simulink model "pi_OfflineRL_H2DF_2023a"  (R2023a)
settings: Solver=FixedStepAuto  StartTime=0.0  StopTime=inf  FixedStep=0.001  RelTol=1e-3  EnableMultiTasking=on
values from neighbouring files (symbols this model uses):
  C2C_NMPC = init_C2C_NMPC_H2DF(C2C_NMPC.expdata)    [init_pi_OfflineRL_H2DF_2023a.m]
  LowerLimit = ([0.17e-3;350;-2;2e-3] - C2C_NMPC.Normalization.controls.mean)./(C2C_NMPC.Normalization.controls.std)    [init_pi_OfflineRL_H2DF_2023a.m]
  UpperLimit = ([0.5e-3;900;10;5.5e-3] - C2C_NMPC.Normalization.controls.mean)./(C2C_NMPC.Normalization.controls.std)    [init_pi_OfflineRL_H2DF_2023a.m]
undefined symbols (not defined in the file or in its folder): DiscIntNeverNeededParam
libraries: deeplib x9, rllib x3, raspberrypiNetworklib x1
(part 3 of 4)

== system pi_OfflineRL_H2DF_2023a/main_C2C/main_C2C_RL/RL_Controller/Subsystem ==
  note: 1:TD3
      | 2:PPO
  Refernce : Inport
  Outputs : Inport  Port=2
  Enable : Inport  Port=3
  LSTM States : Inport  Port=4
  If : If
  If Action Subsystem : Subsystem  TreatAsAtomicUnit=on
  If Action Subsystem1 : Subsystem  TreatAsAtomicUnit=on
  Merge : Merge
  Selector3 : Selector  IndexOptions=Index vector (dialog)  Indices=[5:8]  OutputSizes=1
  Observation : Outport
  wires:
  Selector3/1 -> If Action Subsystem/1(Reference)
  LSTM States/1 -> If Action Subsystem/3(LSTM States)
  Refernce/1 -> Selector3/1
  Outputs/1 -> If Action Subsystem/2(Outputs)
  Enable/1 -> If/1
  If/1 -> If Action Subsystem/Action
  If/2 -> If Action Subsystem1/Action
  If Action Subsystem/1(observations) -> Merge/1
  If Action Subsystem1/1(observations) -> Merge/2
  Merge/1 -> Observation/1

== system pi_OfflineRL_H2DF_2023a/main_C2C/main_C2C_RL/post_processing/ denormalizing reference ==
  IMEP_norm : Inport
  NOX_norm : Inport  Port=2
  soot_norm : Inport  Port=3
  MPRR_norm : Inport  Port=4
  Constant : Constant  Value=C2C_NMPC.Normalization.outputs.mean(1)
  Constant1 : Constant  Value=C2C_NMPC.Normalization.outputs.mean(2)
  Constant2 : Constant  Value=C2C_NMPC.Normalization.outputs.mean(3)
  Constant3 : Constant  Value=C2C_NMPC.Normalization.outputs.mean(4)
  Gain : Gain  Gain=C2C_NMPC.Normalization.outputs.std(1)
  Gain1 : Gain  Gain=C2C_NMPC.Normalization.outputs.std(2)
  Gain2 : Gain  Gain=C2C_NMPC.Normalization.outputs.std(3)
  Gain3 : Gain  Gain=C2C_NMPC.Normalization.outputs.std(4)
  Sum{1..3,5} (4 alike) : Sum  Inputs=|++
  IMEP : Outport
  NOX : Outport  Port=2
  soot : Outport  Port=3
  MPRR : Outport  Port=4
  wires:
  Gain/1 -> Sum5/1
  IMEP_norm/1 -> Gain/1
  Constant/1 -> Sum5/2
  Sum5/1 -> IMEP/1
  Gain1/1 -> Sum1/1
  Constant1/1 -> Sum1/2
  NOX_norm/1 -> Gain1/1
  Sum1/1 -> NOX/1
  Gain2/1 -> Sum2/1
  Constant2/1 -> Sum2/2
  soot_norm/1 -> Gain2/1
  Sum2/1 -> soot/1
  Gain3/1 -> Sum3/1
  Constant3/1 -> Sum3/2
  MPRR_norm/1 -> Gain3/1
  Sum3/1 -> MPRR/1

== system pi_OfflineRL_H2DF_2023a/main_C2C/main_C2C_RL/post_processing/Subsystem ==
  controller_ status : Inport
  LSTM_States : Inport  Port=2
  Selector2 : Selector  IndexOptions=Index vector (dialog)  Indices=[1:(C2C_NMPC.Dims.n_hidden_states+ C2C_NMPC.Dims.n_cell_states)]  OutputSizes=1
  Selector3 : Selector  IndexOptions=Index vector (dialog)  Indices=[41:56]  OutputSizes=1
  Subtract : Sum  Inputs=+-
  Out1 : Outport
  wires:
  Selector3/1 -> Subtract/1
  Selector2/1 -> Subtract/2
  controller_ status/1 -> Selector3/1
  Subtract/1 -> Out1/1
  LSTM_States/1 -> Selector2/1

== system pi_OfflineRL_H2DF_2023a/main_C2C/main_C2C_RL/post_processing/Subsystem1 ==
  controller_ status : Inport
  Last_Output_MC : Inport  Port=2
  " denormalizing reference" : Subsystem
  Demux : Demux
  Mux : Mux
  Mux1 : Mux  Inputs=2
  Mux2 : Mux
  Selector1 : Selector  IndexOptions=Index vector (dialog)  Indices=[(4 + C2C_NMPC.Dims.n_controls * C2C_NMPC.Opts.N + 1 * (C2C_NMPC.Dims.n_states) + C2C_NMPC.Dims.n_LSTM_states + C2C_NMPC.Dims.n_controls +1):( 4 + C2C_NMPC.Dims.n_controls * C2C_NMPC.Opts.N + 2* C2C_NMPC.Dims.n_states)]  OutputSizes=1
  Selector2 : Selector  IndexOptions=Index vector (dialog)  Indices=[(4 + C2C_NMPC.Dims.n_controls * C2C_NMPC.Opts.N + 2 * (C2C_NMPC.Dims.n_states) + C2C_NMPC.Dims.n_LSTM_states + C2C_NMPC.Dims.n_controls +1):( 4 + C2C_NMPC.Dims.n_controls * C2C_NMPC.Opts.N + 3* C2C_NMPC.Dims.n_states)]  OutputSizes=1
  Selector3 : Selector  IndexOptions=Index vector (dialog)  Indices=[(4 + C2C_NMPC.Dims.n_controls * C2C_NMPC.Opts.N + 1* (C2C_NMPC.Dims.n_LSTM_states + C2C_NMPC.Dims.n_controls) +1) : (4 + C2C_NMPC.Dims.n_controls * C2C_NMPC.Opts.N + 1* C2C_NMPC.Dims.n_states)]  OutputSizes=1
  Selector4 : Selector  IndexOptions=Index vector (dialog)  Indices=[(4 + C2C_NMPC.Dims.n_controls * C2C_NMPC.Opts.N + 3 * (C2C_NMPC.Dims.n_states) + C2C_NMPC.Dims.n_LSTM_states + C2C_NMPC.Dims.n_controls +1):( 4 + C2C_NMPC.Dims.n_controls * C2C_NMPC.Opts.N + 4* C2C_NMPC.Dims.n_states)]  OutputSizes=1
  Subsystem : Subsystem
  Out1 : Outport
  wires:
  Last_Output_MC/1 -> Demux/1
  controller_ status/1 -> Selector4/1, Selector2/1, Selector1/1, Selector3/1
  Mux1/1 -> Out1/1
  Mux/1 -> Mux1/2
  Demux/1 -> " denormalizing reference"/1(IMEP_norm)
  Demux/2 -> " denormalizing reference"/2(NOX_norm)
  Demux/3 -> " denormalizing reference"/3(soot_norm)
  Demux/4 -> " denormalizing reference"/4(MPRR_norm)
  " denormalizing reference"/2(NOX) -> Mux2/2
  " denormalizing reference"/1(IMEP) -> Mux2/1
  " denormalizing reference"/3(soot) -> Mux2/3
  " denormalizing reference"/4(MPRR) -> Mux2/4
  Mux2/1 -> Mux1/1
  Subsystem/1(Node_0) -> Mux/1
  Selector3/1 -> Subsystem/1(In1)
  Selector1/1 -> Subsystem/2(In2)
  Subsystem/2(Node_1) -> Mux/2
  Subsystem/3(Node_2) -> Mux/3
  Subsystem/4(Node_3) -> Mux/4
  Selector4/1 -> Subsystem/4(In4)
  Selector2/1 -> Subsystem/3(In3)

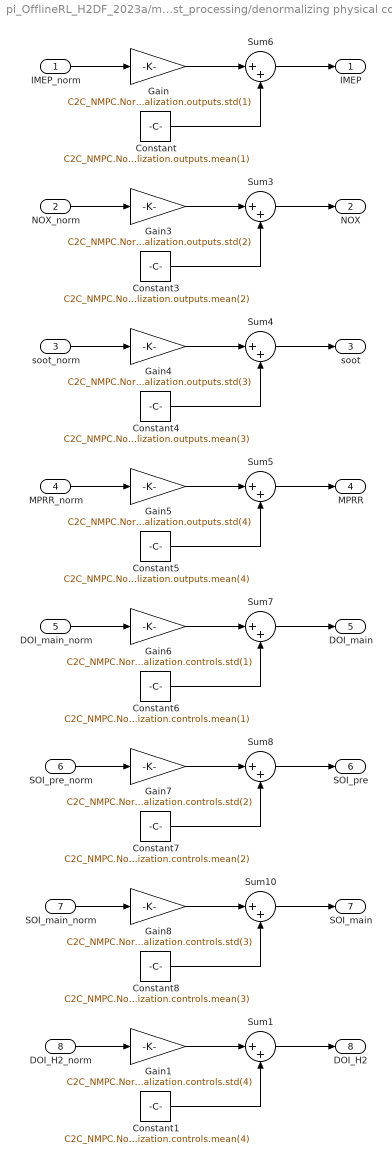
== system pi_OfflineRL_H2DF_2023a/main_C2C/main_C2C_RL/post_processing/denormalizing physical controls and outputs ==
  IMEP_norm : Inport
  NOX_norm : Inport  Port=2
  soot_norm : Inport  Port=3
  MPRR_norm : Inport  Port=4
  DOI_main_norm : Inport  Port=5
  SOI_pre_norm : Inport  Port=6
  SOI_main_norm : Inport  Port=7
  DOI_H2_norm : Inport  Port=8
  Constant : Constant  Value=C2C_NMPC.Normalization.outputs.mean(1)
  Constant1 : Constant  Value=C2C_NMPC.Normalization.controls.mean(4)
  Constant3 : Constant  Value=C2C_NMPC.Normalization.outputs.mean(2)
  Constant4 : Constant  Value=C2C_NMPC.Normalization.outputs.mean(3)
  Constant5 : Constant  Value=C2C_NMPC.Normalization.outputs.mean(4)
  Constant6 : Constant  Value=C2C_NMPC.Normalization.controls.mean(1)
  Constant7 : Constant  Value=C2C_NMPC.Normalization.controls.mean(2)
  Constant8 : Constant  Value=C2C_NMPC.Normalization.controls.mean(3)
  Gain : Gain  Gain=C2C_NMPC.Normalization.outputs.std(1)
  Gain1 : Gain  Gain=C2C_NMPC.Normalization.controls.std(4)
  Gain3 : Gain  Gain=C2C_NMPC.Normalization.outputs.std(2)
  Gain4 : Gain  Gain=C2C_NMPC.Normalization.outputs.std(3)
  Gain5 : Gain  Gain=C2C_NMPC.Normalization.outputs.std(4)
  Gain6 : Gain  Gain=C2C_NMPC.Normalization.controls.std(1)
  Gain7 : Gain  Gain=C2C_NMPC.Normalization.controls.std(2)
  Gain8 : Gain  Gain=C2C_NMPC.Normalization.controls.std(3)
  Sum{1,3..8,10} (8 alike) : Sum  Inputs=|++
  IMEP : Outport
  NOX : Outport  Port=2
  soot : Outport  Port=3
  MPRR : Outport  Port=4
  DOI_main : Outport  Port=5
  SOI_pre : Outport  Port=6
  SOI_main : Outport  Port=7
  DOI_H2 : Outport  Port=8
  wires:
  Gain4/1 -> Sum4/1
  Constant3/1 -> Sum3/2
  Constant4/1 -> Sum4/2
  Gain3/1 -> Sum3/1
  Constant5/1 -> Sum5/2
  Gain5/1 -> Sum5/1
  Constant/1 -> Sum6/2
  Sum3/1 -> NOX/1
  NOX_norm/1 -> Gain3/1
  Sum5/1 -> MPRR/1
  Gain/1 -> Sum6/1
  IMEP_norm/1 -> Gain/1
  Sum6/1 -> IMEP/1
  MPRR_norm/1 -> Gain5/1
  Sum4/1 -> soot/1
  soot_norm/1 -> Gain4/1
  Constant7/1 -> Sum8/2
  Gain8/1 -> Sum10/1
  Constant6/1 -> Sum7/2
  Gain7/1 -> Sum8/1
  Sum10/1 -> SOI_main/1
  DOI_main_norm/1 -> Gain6/1
  Sum7/1 -> DOI_main/1
  Gain6/1 -> Sum7/1
  Sum8/1 -> SOI_pre/1
  Constant8/1 -> Sum10/2
  SOI_main_norm/1 -> Gain8/1
  SOI_pre_norm/1 -> Gain7/1
  Sum1/1 -> DOI_H2/1
  Constant1/1 -> Sum1/2
  Gain1/1 -> Sum1/1
  DOI_H2_norm/1 -> Gain1/1

== system pi_OfflineRL_H2DF_2023a/main_C2C/main_C2C_RL/pre_processing1/normalize_last_outputs_MC ==
  data_in : Inport
  Constant : Constant  Value=C2C_NMPC.Normalization.outputs.mean(1)
  Constant1 : Constant  Value=C2C_NMPC.Normalization.outputs.mean(2)
  Constant2 : Constant  Value=C2C_NMPC.Normalization.outputs.mean(3)
  Constant3 : Constant  Value=C2C_NMPC.Normalization.outputs.mean(4)
  Demux : Demux
  Gain : Gain  Gain=1/C2C_NMPC.Normalization.outputs.std(1)
  Gain1 : Gain  Gain=1/C2C_NMPC.Normalization.outputs.std(2)
  Gain2 : Gain  Gain=1/C2C_NMPC.Normalization.outputs.std(3)
  Gain3 : Gain  Gain=1/C2C_NMPC.Normalization.outputs.std(4)
  Mux : Mux
  Selector1 : Selector  IndexOptions=Index vector (dialog)  Indices=[1:4]  OutputSizes=1
  Sum{1..3,5} (4 alike) : Sum  Inputs=|+-
  last_outputs_MC : Outport  VectorParamsAs1DForOutWhenUnconnected=off
  wires:
  Demux/2 -> Sum1/1
  Constant2/1 -> Sum2/2
  Sum2/1 -> Gain2/1
  Sum1/1 -> Gain1/1
  Gain3/1 -> Mux/4
  Gain1/1 -> Mux/2
  Constant1/1 -> Sum1/2
  Demux/3 -> Sum2/1
  Gain2/1 -> Mux/3
  Mux/1 -> last_outputs_MC/1
  Constant3/1 -> Sum3/2
  Sum3/1 -> Gain3/1
  Gain/1 -> Mux/1
  Sum5/1 -> Gain/1
  Constant/1 -> Sum5/2
  Demux/1 -> Sum5/1
  data_in/1 -> Selector1/1
  Demux/4 -> Sum3/1
  Selector1/1 -> Demux/1

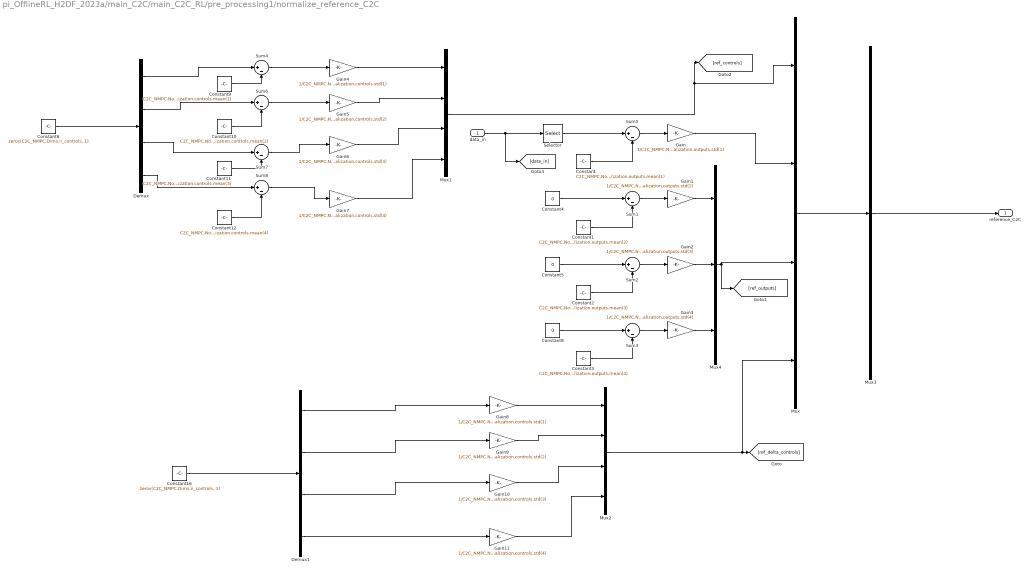
== system pi_OfflineRL_H2DF_2023a/main_C2C/main_C2C_RL/pre_processing1/normalize_reference_C2C ==
  data_in : Inport
  Constant : Constant  Value=C2C_NMPC.Normalization.outputs.mean(1)
  Constant1 : Constant  Value=C2C_NMPC.Normalization.outputs.mean(2)
  Constant10 : Constant  Value=C2C_NMPC.Normalization.controls.mean(2)
  Constant11 : Constant  Value=C2C_NMPC.Normalization.controls.mean(3)
  Constant12 : Constant  Value=C2C_NMPC.Normalization.controls.mean(4)
  Constant16 : Constant  Value=zeros(C2C_NMPC.Dims.n_controls, 1)
  Constant2 : Constant  Value=C2C_NMPC.Normalization.outputs.mean(3)
  Constant3 : Constant  Value=C2C_NMPC.Normalization.outputs.mean(4)
  Constant4 : Constant  Value=0
  Constant5 : Constant  Value=0
  Constant6 : Constant  Value=zeros(C2C_NMPC.Dims.n_controls, 1)
  Constant8 : Constant  Value=0
  Constant9 : Constant  Value=C2C_NMPC.Normalization.controls.mean(1)
  Demux : Demux
  Demux1 : Demux
  Gain : Gain  Gain=1/C2C_NMPC.Normalization.outputs.std(1)
  Gain1 : Gain  Gain=1/C2C_NMPC.Normalization.outputs.std(2)
  Gain10 : Gain  Gain=1/C2C_NMPC.Normalization.controls.std(3)
  Gain11 : Gain  Gain=1/C2C_NMPC.Normalization.controls.std(4)
  Gain2 : Gain  Gain=1/C2C_NMPC.Normalization.outputs.std(3)
  Gain3 : Gain  Gain=1/C2C_NMPC.Normalization.outputs.std(4)
  Gain4 : Gain  Gain=1/C2C_NMPC.Normalization.controls.std(1)
  Gain5 : Gain  Gain=1/C2C_NMPC.Normalization.controls.std(2)
  Gain6 : Gain  Gain=1/C2C_NMPC.Normalization.controls.std(3)
  Gain7 : Gain  Gain=1/C2C_NMPC.Normalization.controls.std(4)
  Gain8 : Gain  Gain=1/C2C_NMPC.Normalization.controls.std(1)
  Gain9 : Gain  Gain=1/C2C_NMPC.Normalization.controls.std(2)
  Mux : Mux
  Mux1 : Mux
  Mux2 : Mux
  Mux3 : Mux  Inputs=1
  Mux4 : Mux  Inputs=3
  Selector : Selector  IndexOptions=Index vector (dialog)  Indices=[5]  OutputSizes=1
  Sum{1..8} (8 alike) : Sum  Inputs=|+-
  reference_C2C : Outport  VectorParamsAs1DForOutWhenUnconnected=off
  wires:
  Constant/1 -> Sum5/2
  data_in/1 -> [data_in], Selector/1
  Sum5/1 -> Gain/1
  Selector/1 -> Sum5/1
  Constant4/1 -> Sum1/1
  Sum1/1 -> Gain1/1
  Constant1/1 -> Sum1/2
  Constant5/1 -> Sum2/1
  Sum2/1 -> Gain2/1
  Constant2/1 -> Sum2/2
  Constant8/1 -> Sum3/1
  Sum3/1 -> Gain3/1
  Constant3/1 -> Sum3/2
  Demux/1 -> Sum4/1
  Sum4/1 -> Gain4/1
  Constant9/1 -> Sum4/2
  Constant6/1 -> Demux/1
  Demux/2 -> Sum6/1
  Constant10/1 -> Sum6/2
  Sum6/1 -> Gain5/1
  Gain5/1 -> Mux1/2
  Gain4/1 -> Mux1/1
  Sum7/1 -> Gain6/1
  Constant11/1 -> Sum7/2
  Demux/3 -> Sum7/1
  Constant12/1 -> Sum8/2
  Sum8/1 -> Gain7/1
  Demux/4 -> Sum8/1
  Gain7/1 -> Mux1/4
  Gain6/1 -> Mux1/3
  Gain9/1 -> Mux2/2
  Gain11/1 -> Mux2/4
  Constant16/1 -> Demux1/1
  Gain8/1 -> Mux2/1
  Gain10/1 -> Mux2/3
  Demux1/4 -> Gain11/1
  Demux1/3 -> Gain10/1
  Demux1/2 -> Gain9/1
  Demux1/1 -> Gain8/1
  Mux2/1 -> [ref_delta_controls], Mux/4
  Mux3/1 -> reference_C2C/1
  Mux/1 -> Mux3/1
  Gain1/1 -> Mux4/1
  Gain2/1 -> Mux4/2
  Gain3/1 -> Mux4/3
  Gain/1 -> Mux/2
  Mux4/1 -> Mux/3, [ref_outputs]
  Mux1/1 -> [ref_controls], Mux/1

== system pi_OfflineRL_H2DF_2023a/main_C2C_RL/RL_Controller/RL_Controller_ifAction/RL_Controller_PPO1 ==
  In : Inport
  Action Port : ActionPort  ActionPortLabel=case [ 3 ]:
  Data Type Conversion1 : DataTypeConversion  OutDataTypeStr=single  SaturateOnIntegerOverflow=off  RndMeth=Floor
  Predict1 : deeplib/Predict  Network=Network from MAT-file  NetworkFunction=squeezenet  NetworkFilePath=C:\GIT\sharma_ma_rlonh2df\acados_implementation\rl\Results\20240912\Agent.mat  MiniBatchSize=128  InputDataFormats={ 'input_1', 'BC' }  Predictions=on  Activations={}  ForceInterpretedSim=off  EnableDLNetwork=on
  Reshape : Reshape  OutputDimensionality=Row vector (2-D)
  Selector1 : Selector  IndexOptions=Index vector (dialog)  Indices=[13:16]  OutputSizes=1
  Selector2 : Selector  IndexOptions=Index vector (dialog)  Indices=[17:24]  OutputSizes=1
  Selector3 : Selector  IndexOptions=Index vector (dialog)  Indices=[1:12]  OutputSizes=1
  Selector4 : Selector  IndexOptions=Index vector (dialog)  Indices=[25]  OutputSizes=1
  Subsystem : Subsystem
  Control_norm_NN_params : Outport
  wires:
  Predict1/1 -> Control_norm_NN_params/1
  Reshape/1 -> Predict1/1
  Data Type Conversion1/1 -> Reshape/1
  Subsystem/1(Observation) -> Data Type Conversion1/1
  In/1 -> Selector3/1, Selector1/1, Selector4/1, Selector2/1
  Selector3/1 -> Subsystem/1(Refernce)
  Selector1/1 -> Subsystem/2(Outputs)
  Selector2/1 -> Subsystem/3(LSTM States)
  Selector4/1 -> Subsystem/4(Enable)

== system pi_OfflineRL_H2DF_2023a/main_C2C_RL/RL_Controller/RL_Controller_ifAction/RL_Controller_PPO2 ==
  In : Inport
  Action Port : ActionPort  ActionPortLabel=case [ 4 ]:
  Data Type Conversion1 : DataTypeConversion  OutDataTypeStr=single  SaturateOnIntegerOverflow=off  RndMeth=Floor
  Predict1 : deeplib/Predict  Network=Network from MAT-file  NetworkFunction=squeezenet  NetworkFilePath=C:\GIT\sharma_ma_rlonh2df\acados_implementation\rl\Results\2024095\Agent.mat  MiniBatchSize=128  InputDataFormats={ 'input_1', 'BC' }  Predictions=on  Activations={}  ForceInterpretedSim=off  EnableDLNetwork=on
  Reshape : Reshape  OutputDimensionality=Row vector (2-D)
  Selector1 : Selector  IndexOptions=Index vector (dialog)  Indices=[13:16]  OutputSizes=1
  Selector2 : Selector  IndexOptions=Index vector (dialog)  Indices=[17:24]  OutputSizes=1
  Selector3 : Selector  IndexOptions=Index vector (dialog)  Indices=[1:12]  OutputSizes=1
  Selector4 : Selector  IndexOptions=Index vector (dialog)  Indices=[25]  OutputSizes=1
  Subsystem : Subsystem
  Control_norm_NN_params : Outport
  wires:
  Predict1/1 -> Control_norm_NN_params/1
  Reshape/1 -> Predict1/1
  Data Type Conversion1/1 -> Reshape/1
  Subsystem/1(Observation) -> Data Type Conversion1/1
  In/1 -> Selector3/1, Selector1/1, Selector4/1, Selector2/1
  Selector3/1 -> Subsystem/1(Refernce)
  Selector1/1 -> Subsystem/2(Outputs)
  Selector2/1 -> Subsystem/3(LSTM States)
  Selector4/1 -> Subsystem/4(Enable)

== system pi_OfflineRL_H2DF_2023a/main_C2C_RL/RL_Controller/RL_Controller_ifAction/RL_Controller_PPO3 ==
  In : Inport
  Action Port : ActionPort  ActionPortLabel=case [ 5 ]:
  Data Type Conversion1 : DataTypeConversion  OutDataTypeStr=single  SaturateOnIntegerOverflow=off  RndMeth=Floor
  Predict1 : deeplib/Predict  Network=Network from MAT-file  NetworkFunction=squeezenet  NetworkFilePath=C:\GIT\sharma_ma_rlonh2df\acados_implementation\rl\Results\2024097\Agent.mat  MiniBatchSize=128  InputDataFormats={ 'input_1', 'BC' }  Predictions=on  Activations={}  ForceInterpretedSim=off  EnableDLNetwork=on
  Reshape : Reshape  OutputDimensionality=Row vector (2-D)
  Selector1 : Selector  IndexOptions=Index vector (dialog)  Indices=[13:16]  OutputSizes=1
  Selector2 : Selector  IndexOptions=Index vector (dialog)  Indices=[17:24]  OutputSizes=1
  Selector3 : Selector  IndexOptions=Index vector (dialog)  Indices=[1:12]  OutputSizes=1
  Selector4 : Selector  IndexOptions=Index vector (dialog)  Indices=[25]  OutputSizes=1
  Subsystem : Subsystem
  Control_norm_NN_params : Outport
  wires:
  Predict1/1 -> Control_norm_NN_params/1
  Reshape/1 -> Predict1/1
  Data Type Conversion1/1 -> Reshape/1
  Subsystem/1(Observation) -> Data Type Conversion1/1
  In/1 -> Selector3/1, Selector1/1, Selector4/1, Selector2/1
  Selector3/1 -> Subsystem/1(Refernce)
  Selector1/1 -> Subsystem/2(Outputs)
  Selector2/1 -> Subsystem/3(LSTM States)
  Selector4/1 -> Subsystem/4(Enable)

== system pi_OfflineRL_H2DF_2023a/main_C2C_RL/RL_Controller/RL_Controller_ifAction/RL_Controller_PPO4 ==
  In : Inport
  Action Port : ActionPort  ActionPortLabel=case [ 6 ]:
  Data Type Conversion1 : DataTypeConversion  OutDataTypeStr=single  SaturateOnIntegerOverflow=off  RndMeth=Floor
  Predict1 : deeplib/Predict  Network=Network from MAT-file  NetworkFunction=squeezenet  NetworkFilePath=C:\GIT\sharma_ma_rlonh2df\acados_implementation\rl\Results\2024098\Agent.mat  MiniBatchSize=128  InputDataFormats={ 'input_1', 'BC' }  Predictions=on  Activations={}  ForceInterpretedSim=off  EnableDLNetwork=on
  Reshape : Reshape  OutputDimensionality=Row vector (2-D)
  Selector1 : Selector  IndexOptions=Index vector (dialog)  Indices=[13:16]  OutputSizes=1
  Selector2 : Selector  IndexOptions=Index vector (dialog)  Indices=[17:24]  OutputSizes=1
  Selector3 : Selector  IndexOptions=Index vector (dialog)  Indices=[1:12]  OutputSizes=1
  Selector4 : Selector  IndexOptions=Index vector (dialog)  Indices=[25]  OutputSizes=1
  Subsystem : Subsystem
  Control_norm_NN_params : Outport
  wires:
  Predict1/1 -> Control_norm_NN_params/1
  Reshape/1 -> Predict1/1
  Data Type Conversion1/1 -> Reshape/1
  Subsystem/1(Observation) -> Data Type Conversion1/1
  In/1 -> Selector3/1, Selector1/1, Selector4/1, Selector2/1
  Selector3/1 -> Subsystem/1(Refernce)
  Selector1/1 -> Subsystem/2(Outputs)
  Selector2/1 -> Subsystem/3(LSTM States)
  Selector4/1 -> Subsystem/4(Enable)

== system pi_OfflineRL_H2DF_2023a/main_C2C_RL/RL_Controller/RL_Controller_ifAction/RL_Controller_PPO5 ==
  In : Inport
  Action Port : ActionPort  ActionPortLabel=case [ 1 ]:
  Data Type Conversion1 : DataTypeConversion  OutDataTypeStr=single  SaturateOnIntegerOverflow=off  RndMeth=Floor
  Predict1 : deeplib/Predict  Network=Network from MAT-file  NetworkFunction=squeezenet  NetworkFilePath=C:\GIT\sharma_ma_rlonh2df\acados_implementation\rl\Results\20240909\Agent.mat  MiniBatchSize=128  InputDataFormats={ 'input_1', 'BC' }  Predictions=on  Activations={}  ForceInterpretedSim=off  EnableDLNetwork=on
  Reshape : Reshape  OutputDimensionality=Row vector (2-D)
  Selector1 : Selector  IndexOptions=Index vector (dialog)  Indices=[13:16]  OutputSizes=1
  Selector2 : Selector  IndexOptions=Index vector (dialog)  Indices=[17:24]  OutputSizes=1
  Selector3 : Selector  IndexOptions=Index vector (dialog)  Indices=[1:12]  OutputSizes=1
  Selector4 : Selector  IndexOptions=Index vector (dialog)  Indices=[25]  OutputSizes=1
  Subsystem : Subsystem
  Control_norm_NN_params : Outport
  wires:
  Predict1/1 -> Control_norm_NN_params/1
  Reshape/1 -> Predict1/1
  Data Type Conversion1/1 -> Reshape/1
  Subsystem/1(Observation) -> Data Type Conversion1/1
  In/1 -> Selector3/1, Selector1/1, Selector4/1, Selector2/1
  Selector3/1 -> Subsystem/1(Refernce)
  Selector1/1 -> Subsystem/2(Outputs)
  Selector2/1 -> Subsystem/3(LSTM States)
  Selector4/1 -> Subsystem/4(Enable)

== system pi_OfflineRL_H2DF_2023a/main_C2C_RL/RL_Controller/RL_Controller_ifAction/RL_Controller_PPO6 ==
  In : Inport
  Action Port : ActionPort  ActionPortLabel=case [ 2 ]:
  Data Type Conversion1 : DataTypeConversion  OutDataTypeStr=single  SaturateOnIntegerOverflow=off  RndMeth=Floor
  Predict1 : deeplib/Predict  Network=Network from MAT-file  NetworkFunction=squeezenet  NetworkFilePath=C:\GIT\sharma_ma_rlonh2df\acados_implementation\rl\Results\20240910\Agent.mat  MiniBatchSize=128  InputDataFormats={ 'input_1', 'BC' }  Predictions=on  Activations={}  ForceInterpretedSim=off  EnableDLNetwork=on
  Reshape : Reshape  OutputDimensionality=Row vector (2-D)
  Selector1 : Selector  IndexOptions=Index vector (dialog)  Indices=[13:16]  OutputSizes=1
  Selector2 : Selector  IndexOptions=Index vector (dialog)  Indices=[17:24]  OutputSizes=1
  Selector3 : Selector  IndexOptions=Index vector (dialog)  Indices=[1:12]  OutputSizes=1
  Selector4 : Selector  IndexOptions=Index vector (dialog)  Indices=[25]  OutputSizes=1
  Subsystem : Subsystem
  Control_norm_NN_params : Outport
  wires:
  Predict1/1 -> Control_norm_NN_params/1
  Reshape/1 -> Predict1/1
  Data Type Conversion1/1 -> Reshape/1
  Subsystem/1(Observation) -> Data Type Conversion1/1
  In/1 -> Selector3/1, Selector1/1, Selector4/1, Selector2/1
  Selector3/1 -> Subsystem/1(Refernce)
  Selector1/1 -> Subsystem/2(Outputs)
  Selector2/1 -> Subsystem/3(LSTM States)
  Selector4/1 -> Subsystem/4(Enable)

== system pi_OfflineRL_H2DF_2023a/main_C2C_RL/RL_Controller/RL_Controller_ifAction/RL_Controller_PPO7 ==
  In : Inport
  Action Port : ActionPort  ActionPortLabel=case [ 7 ]:
  Data Type Conversion1 : DataTypeConversion  OutDataTypeStr=single  SaturateOnIntegerOverflow=off  RndMeth=Floor
  Predict1 : deeplib/Predict  Network=Network from MAT-file  NetworkFunction=squeezenet  NetworkFilePath=C:\GIT\sharma_ma_rlonh2df\acados_implementation\rl\Results\20240913\Agent.mat  MiniBatchSize=128  InputDataFormats={ 'input_1', 'BC' }  Predictions=on  Activations={}  ForceInterpretedSim=off  EnableDLNetwork=on
  Reshape : Reshape  OutputDimensionality=Row vector (2-D)
  Selector1 : Selector  IndexOptions=Index vector (dialog)  Indices=[13:16]  OutputSizes=1
  Selector2 : Selector  IndexOptions=Index vector (dialog)  Indices=[17:24]  OutputSizes=1
  Selector3 : Selector  IndexOptions=Index vector (dialog)  Indices=[1:12]  OutputSizes=1
  Selector4 : Selector  IndexOptions=Index vector (dialog)  Indices=[25]  OutputSizes=1
  Subsystem : Subsystem
  Control_norm_NN_params : Outport
  wires:
  Predict1/1 -> Control_norm_NN_params/1
  Reshape/1 -> Predict1/1
  Data Type Conversion1/1 -> Reshape/1
  Subsystem/1(Observation) -> Data Type Conversion1/1
  In/1 -> Selector3/1, Selector1/1, Selector4/1, Selector2/1
  Selector3/1 -> Subsystem/1(Refernce)
  Selector1/1 -> Subsystem/2(Outputs)
  Selector2/1 -> Subsystem/3(LSTM States)
  Selector4/1 -> Subsystem/4(Enable)

== system pi_OfflineRL_H2DF_2023a/main_C2C_RL/RL_Controller/RL_Controller_ifAction/RL_Controller_PPO8 ==
  In : Inport
  Action Port : ActionPort  ActionPortLabel=case [ 8 ]:
  Data Type Conversion1 : DataTypeConversion  OutDataTypeStr=single  SaturateOnIntegerOverflow=off  RndMeth=Floor
  Predict1 : deeplib/Predict  Network=Network from MAT-file  NetworkFunction=squeezenet  NetworkFilePath=C:\GIT\sharma_ma_rlonh2df\acados_implementation\rl\Results\20240915\Agent.mat  MiniBatchSize=128  InputDataFormats={ 'input_1', 'BC' }  Predictions=on  Activations={}  ForceInterpretedSim=off  EnableDLNetwork=on
  Reshape : Reshape  OutputDimensionality=Row vector (2-D)
  Selector1 : Selector  IndexOptions=Index vector (dialog)  Indices=[13:16]  OutputSizes=1
  Selector2 : Selector  IndexOptions=Index vector (dialog)  Indices=[17:24]  OutputSizes=1
  Selector3 : Selector  IndexOptions=Index vector (dialog)  Indices=[1:12]  OutputSizes=1
  Selector4 : Selector  IndexOptions=Index vector (dialog)  Indices=[25]  OutputSizes=1
  Subsystem : Subsystem
  Control_norm_NN_params : Outport
  wires:
  Predict1/1 -> Control_norm_NN_params/1
  Reshape/1 -> Predict1/1
  Data Type Conversion1/1 -> Reshape/1
  Subsystem/1(Observation) -> Data Type Conversion1/1
  In/1 -> Selector3/1, Selector1/1, Selector4/1, Selector2/1
  Selector3/1 -> Subsystem/1(Refernce)
  Selector1/1 -> Subsystem/2(Outputs)
  Selector2/1 -> Subsystem/3(LSTM States)
  Selector4/1 -> Subsystem/4(Enable)

== system pi_OfflineRL_H2DF_2023a/main_C2C_RL/RL_Controller/State_Augmentation/Denorm_plant_IMEP_ref1 ==
  outputs : Inport
  Constant : Constant  Value=C2C_NMPC.Normalization.outputs.mean(1)
  Gain : Gain  Gain=C2C_NMPC.Normalization.outputs.std(1)
  Sum6 : Sum  Inputs=|++
  RefIn : Outport
  wires:
  Constant/1 -> Sum6/2
  Gain/1 -> Sum6/1
  Sum6/1 -> RefIn/1
  outputs/1 -> Gain/1  "IMEP"

== system pi_OfflineRL_H2DF_2023a/main_C2C_RL/RL_Controller/State_Augmentation/dyn_H2DF ==
  controls : Inport
  last_outputs : Inport  Port=2
  last_LSTM_states : Inport  Port=3
  dyn_H2DF : MATLAB Function  TreatAsAtomicUnit=on
  outputs : Outport
  LSTM_states : Outport  Port=2
  wires:
  dyn_H2DF/1(outputs) -> outputs/1
  controls/1 -> dyn_H2DF/2(controls)
  last_outputs/1 -> dyn_H2DF/3(last_outputs)
  dyn_H2DF/2(LSTM_states) -> LSTM_states/1
  last_LSTM_states/1 -> dyn_H2DF/1(last_LSTM_states)

== system pi_OfflineRL_H2DF_2023a/main_C2C_RL/RL_Controller/State_Augmentation/dyn_H2DF_state_augmentation ==
  last_LSTM_states : Inport
  controls : Inport  Port=2
  last_outputs : Inport  Port=3
  dyn_H2DF_state_augmentation : MATLAB Function  TreatAsAtomicUnit=on
  LSTM_states : Outport
  wires:
  dyn_H2DF_state_augmentation/1(LSTM_states) -> LSTM_states/1
  last_outputs/1 -> dyn_H2DF_state_augmentation/3(last_outputs)
  last_LSTM_states/1 -> dyn_H2DF_state_augmentation/1(last_LSTM_states)
  controls/1 -> dyn_H2DF_state_augmentation/2(controls)

== system pi_OfflineRL_H2DF_2023a/main_C2C_RL/RL_Controller/Subsystem1/If Action Subsystem ==
  Action Port : ActionPort  ActionPortLabel=if(u1 > 4.5e5)
  Constant : Constant  Value=4
  Out1 : Outport
  wires:
  Constant/1 -> Out1/1

== system pi_OfflineRL_H2DF_2023a/main_C2C_RL/RL_Controller/Subsystem1/If Action Subsystem1 ==
  Action Port : ActionPort  ActionPortLabel=else
  Constant : Constant  Value=2
  Out1 : Outport
  wires:
  Constant/1 -> Out1/1

== system pi_OfflineRL_H2DF_2023a/main_C2C_RL/post_processing/Subsystem1/ denormalizing reference ==
  IMEP_norm : Inport
  NOX_norm : Inport  Port=2
  soot_norm : Inport  Port=3
  MPRR_norm : Inport  Port=4
  Constant : Constant  Value=C2C_NMPC.Normalization.outputs.mean(1)
  Constant1 : Constant  Value=C2C_NMPC.Normalization.outputs.mean(2)
  Constant2 : Constant  Value=C2C_NMPC.Normalization.outputs.mean(3)
  Constant3 : Constant  Value=C2C_NMPC.Normalization.outputs.mean(4)
  Gain : Gain  Gain=C2C_NMPC.Normalization.outputs.std(1)
  Gain1 : Gain  Gain=C2C_NMPC.Normalization.outputs.std(2)
  Gain2 : Gain  Gain=C2C_NMPC.Normalization.outputs.std(3)
  Gain3 : Gain  Gain=C2C_NMPC.Normalization.outputs.std(4)
  Sum{1..3,5} (4 alike) : Sum  Inputs=|++
  IMEP : Outport
  NOX : Outport  Port=2
  soot : Outport  Port=3
  MPRR : Outport  Port=4
  wires:
  Gain/1 -> Sum5/1
  IMEP_norm/1 -> Gain/1
  Constant/1 -> Sum5/2
  Sum5/1 -> IMEP/1
  Gain1/1 -> Sum1/1
  Constant1/1 -> Sum1/2
  NOX_norm/1 -> Gain1/1
  Sum1/1 -> NOX/1
  Gain2/1 -> Sum2/1
  Constant2/1 -> Sum2/2
  soot_norm/1 -> Gain2/1
  Sum2/1 -> soot/1
  Gain3/1 -> Sum3/1
  Constant3/1 -> Sum3/2
  MPRR_norm/1 -> Gain3/1
  Sum3/1 -> MPRR/1

== system pi_OfflineRL_H2DF_2023a/main_C2C_RL/post_processing/Subsystem1/Subsystem ==
  In1 : Inport
  In2 : Inport  Port=2
  In3 : Inport  Port=3
  In4 : Inport  Port=4
  " denormalizing reference1" : Subsystem
  " denormalizing reference2" : Subsystem
  " denormalizing reference3" : Subsystem
  " denormalizing reference4" : Subsystem
  Demux{,1..3} (4 alike) : Demux
  Mux{,1..3} (4 alike) : Mux
  Node_0 : Outport
  Node_1 : Outport  Port=2
  Node_2 : Outport  Port=3
  Node_3 : Outport  Port=4
  wires:
  Demux/1 -> " denormalizing reference1"/1(IMEP_norm)
  Demux/2 -> " denormalizing reference1"/2(NOX_norm)
  Demux/3 -> " denormalizing reference1"/3(soot_norm)
  Demux/4 -> " denormalizing reference1"/4(MPRR_norm)
  In1/1 -> Demux/1
  " denormalizing reference1"/1(IMEP) -> Mux/1
  " denormalizing reference1"/2(NOX) -> Mux/2
  " denormalizing reference1"/3(soot) -> Mux/3
  " denormalizing reference1"/4(MPRR) -> Mux/4
  " denormalizing reference2"/3(soot) -> Mux1/3
  Demux1/3 -> " denormalizing reference2"/3(soot_norm)
  In2/1 -> Demux1/1
  " denormalizing reference2"/2(NOX) -> Mux1/2
  " denormalizing reference2"/1(IMEP) -> Mux1/1
  Demux1/1 -> " denormalizing reference2"/1(IMEP_norm)
  Demux1/4 -> " denormalizing reference2"/4(MPRR_norm)
  Demux1/2 -> " denormalizing reference2"/2(NOX_norm)
  " denormalizing reference2"/4(MPRR) -> Mux1/4
  " denormalizing reference3"/3(soot) -> Mux2/3
  Demux2/3 -> " denormalizing reference3"/3(soot_norm)
  In3/1 -> Demux2/1
  " denormalizing reference3"/2(NOX) -> Mux2/2
  " denormalizing reference3"/1(IMEP) -> Mux2/1
  Demux2/1 -> " denormalizing reference3"/1(IMEP_norm)
  Demux2/4 -> " denormalizing reference3"/4(MPRR_norm)
  Demux2/2 -> " denormalizing reference3"/2(NOX_norm)
  " denormalizing reference3"/4(MPRR) -> Mux2/4
  " denormalizing reference4"/3(soot) -> Mux3/3
  Demux3/3 -> " denormalizing reference4"/3(soot_norm)
  In4/1 -> Demux3/1
  " denormalizing reference4"/2(NOX) -> Mux3/2
  " denormalizing reference4"/1(IMEP) -> Mux3/1
  Demux3/1 -> " denormalizing reference4"/1(IMEP_norm)
  Demux3/4 -> " denormalizing reference4"/4(MPRR_norm)
  Demux3/2 -> " denormalizing reference4"/2(NOX_norm)
  " denormalizing reference4"/4(MPRR) -> Mux3/4
  Mux/1 -> Node_0/1
  Mux1/1 -> Node_1/1
  Mux2/1 -> Node_2/1
  Mux3/1 -> Node_3/1

== system pi_OfflineRL_H2DF_2023a/main_C2C/main_C2C_RL/RL_Controller/RL_Controller_ifAction/RL_Controller_PPO ==
  Obs : Inport
  Action Port : ActionPort
  Policy3 : rllib/Policy  MATFile=C:\GIT\sharma_ma_rlonh2df\acados_implementation\rl\Results\20240823\blockAgentData.mat  SimUsingCodegen=off
  Control_norm_NN_params : Outport
  wires:
  Policy3/1 -> Control_norm_NN_params/1
  Obs/1 -> Policy3/1

== system pi_OfflineRL_H2DF_2023a/main_C2C/main_C2C_RL/RL_Controller/RL_Controller_ifAction/RL_Controller_PPO1 ==
  Obs : Inport
  Action Port : ActionPort
  Constant : Constant  Value=zeros(16,1)
  Policy5 : rllib/Policy  MATFile=C:\GIT\sharma_ma_rlonh2df\acados_implementation\rl\Results\20240818\blockAgentData.mat  SimUsingCodegen=off
  Predict1 : deeplib/Predict  Network=Network from MAT-file  NetworkFunction=squeezenet  NetworkFilePath=C:\GIT\sharma_ma_rlonh2df\acados_implementation\rl\Results\20240818\model.mat  MiniBatchSize=128  InputDataFormats={ 'input_1', 'BC' }  Predictions=on  Activations={}  ForceInterpretedSim=off  EnableDLNetwork=on
  Reshape : Reshape  OutputDimensionality=Row vector (2-D)
  Control_norm_NN_params : Outport
  wires:
  Policy5/1 -> Control_norm_NN_params/1
  Obs/1 -> Reshape/1, Policy5/1
  Reshape/1 -> Predict1/1

== system pi_OfflineRL_H2DF_2023a/main_C2C/main_C2C_RL/RL_Controller/RL_Controller_ifAction/RL_Controller_TD3 ==
  Obs : Inport
  Action Port : ActionPort
  Policy3 : rllib/Policy  MATFile=C:\GIT\sharma_ma_rlonh2df\acados_implementation\rl\Results\20240823\blockAgentData.mat  SimUsingCodegen=off
  Scope : Scope
  Control_norm_NN_params : Outport
  wires:
  Policy3/1 -> Control_norm_NN_params/1
  Obs/1 -> Policy3/1

== system pi_OfflineRL_H2DF_2023a/main_C2C/main_C2C_RL/RL_Controller/State_Augmentation/Denorm_plant_IMEP_ref1 ==
  outputs : Inport
  Constant : Constant  Value=C2C_NMPC.Normalization.outputs.mean(1)
  Gain : Gain  Gain=C2C_NMPC.Normalization.outputs.std(1)
  Sum6 : Sum  Inputs=|++
  RefIn : Outport
  wires:
  Constant/1 -> Sum6/2
  Gain/1 -> Sum6/1
  Sum6/1 -> RefIn/1
  outputs/1 -> Gain/1  "IMEP"

== system pi_OfflineRL_H2DF_2023a/main_C2C/main_C2C_RL/RL_Controller/State_Augmentation/dyn_H2DF ==
  controls : Inport
  last_outputs : Inport  Port=2
  last_LSTM_states : Inport  Port=3
  dyn_H2DF : MATLAB Function  TreatAsAtomicUnit=on
  outputs : Outport
  LSTM_states : Outport  Port=2
  wires:
  dyn_H2DF/1(outputs) -> outputs/1
  controls/1 -> dyn_H2DF/2(controls)
  last_outputs/1 -> dyn_H2DF/3(last_outputs)
  dyn_H2DF/2(LSTM_states) -> LSTM_states/1
  last_LSTM_states/1 -> dyn_H2DF/1(last_LSTM_states)

== system pi_OfflineRL_H2DF_2023a/main_C2C/main_C2C_RL/RL_Controller/State_Augmentation/dyn_H2DF_state_augmentation ==
  last_LSTM_states : Inport
  controls : Inport  Port=2
  last_outputs : Inport  Port=3
  dyn_H2DF_state_augmentation : MATLAB Function  TreatAsAtomicUnit=on
  LSTM_states : Outport
  wires:
  dyn_H2DF_state_augmentation/1(LSTM_states) -> LSTM_states/1
  last_outputs/1 -> dyn_H2DF_state_augmentation/3(last_outputs)
  last_LSTM_states/1 -> dyn_H2DF_state_augmentation/1(last_LSTM_states)
  controls/1 -> dyn_H2DF_state_augmentation/2(controls)

== system pi_OfflineRL_H2DF_2023a/main_C2C/main_C2C_RL/RL_Controller/Subsystem/If Action Subsystem ==
  Reference : Inport
  Outputs : Inport  Port=2
  LSTM States : Inport  Port=3
  Action Port : ActionPort
  generate observations : Subsystem
  observations : Outport
  wires:
  LSTM States/1 -> generate observations/3(LSTM States)
  Reference/1 -> generate observations/2(Reference)
  generate observations/1(observations) -> observations/1
  Outputs/1 -> generate observations/1(Outputs)

== system pi_OfflineRL_H2DF_2023a/main_C2C/main_C2C_RL/RL_Controller/Subsystem/If Action Subsystem1 ==
  Action Port : ActionPort
  Constant : Constant  Value=zeros(16,1)
  observations : Outport
  wires:
  Constant/1 -> observations/1

== system pi_OfflineRL_H2DF_2023a/main_C2C/main_C2C_RL/post_processing/Subsystem1/ denormalizing reference ==
  IMEP_norm : Inport
  NOX_norm : Inport  Port=2
  soot_norm : Inport  Port=3
  MPRR_norm : Inport  Port=4
  Constant : Constant  Value=C2C_NMPC.Normalization.outputs.mean(1)
  Constant1 : Constant  Value=C2C_NMPC.Normalization.outputs.mean(2)
  Constant2 : Constant  Value=C2C_NMPC.Normalization.outputs.mean(3)
  Constant3 : Constant  Value=C2C_NMPC.Normalization.outputs.mean(4)
  Gain : Gain  Gain=C2C_NMPC.Normalization.outputs.std(1)
  Gain1 : Gain  Gain=C2C_NMPC.Normalization.outputs.std(2)
  Gain2 : Gain  Gain=C2C_NMPC.Normalization.outputs.std(3)
  Gain3 : Gain  Gain=C2C_NMPC.Normalization.outputs.std(4)
  Sum{1..3,5} (4 alike) : Sum  Inputs=|++
  IMEP : Outport
  NOX : Outport  Port=2
  soot : Outport  Port=3
  MPRR : Outport  Port=4
  wires:
  Gain/1 -> Sum5/1
  IMEP_norm/1 -> Gain/1
  Constant/1 -> Sum5/2
  Sum5/1 -> IMEP/1
  Gain1/1 -> Sum1/1
  Constant1/1 -> Sum1/2
  NOX_norm/1 -> Gain1/1
  Sum1/1 -> NOX/1
  Gain2/1 -> Sum2/1
  Constant2/1 -> Sum2/2
  soot_norm/1 -> Gain2/1
  Sum2/1 -> soot/1
  Gain3/1 -> Sum3/1
  Constant3/1 -> Sum3/2
  MPRR_norm/1 -> Gain3/1
  Sum3/1 -> MPRR/1

== system pi_OfflineRL_H2DF_2023a/main_C2C/main_C2C_RL/post_processing/Subsystem1/Subsystem ==
  In1 : Inport
  In2 : Inport  Port=2
  In3 : Inport  Port=3
  In4 : Inport  Port=4
  " denormalizing reference1" : Subsystem
  " denormalizing reference2" : Subsystem
  " denormalizing reference3" : Subsystem
  " denormalizing reference4" : Subsystem
  Demux{,1..3} (4 alike) : Demux
  Mux{,1..3} (4 alike) : Mux
  Node_0 : Outport
  Node_1 : Outport  Port=2
  Node_2 : Outport  Port=3
  Node_3 : Outport  Port=4
  wires:
  Demux/1 -> " denormalizing reference1"/1(IMEP_norm)
  Demux/2 -> " denormalizing reference1"/2(NOX_norm)
  Demux/3 -> " denormalizing reference1"/3(soot_norm)
  Demux/4 -> " denormalizing reference1"/4(MPRR_norm)
  In1/1 -> Demux/1
  " denormalizing reference1"/1(IMEP) -> Mux/1
  " denormalizing reference1"/2(NOX) -> Mux/2
  " denormalizing reference1"/3(soot) -> Mux/3
  " denormalizing reference1"/4(MPRR) -> Mux/4
  " denormalizing reference2"/3(soot) -> Mux1/3
  Demux1/3 -> " denormalizing reference2"/3(soot_norm)
  In2/1 -> Demux1/1
  " denormalizing reference2"/2(NOX) -> Mux1/2
  " denormalizing reference2"/1(IMEP) -> Mux1/1
  Demux1/1 -> " denormalizing reference2"/1(IMEP_norm)
  Demux1/4 -> " denormalizing reference2"/4(MPRR_norm)
  Demux1/2 -> " denormalizing reference2"/2(NOX_norm)
  " denormalizing reference2"/4(MPRR) -> Mux1/4
  " denormalizing reference3"/3(soot) -> Mux2/3
  Demux2/3 -> " denormalizing reference3"/3(soot_norm)
  In3/1 -> Demux2/1
  " denormalizing reference3"/2(NOX) -> Mux2/2
  " denormalizing reference3"/1(IMEP) -> Mux2/1
  Demux2/1 -> " denormalizing reference3"/1(IMEP_norm)
  Demux2/4 -> " denormalizing reference3"/4(MPRR_norm)
  Demux2/2 -> " denormalizing reference3"/2(NOX_norm)
  " denormalizing reference3"/4(MPRR) -> Mux2/4
  " denormalizing reference4"/3(soot) -> Mux3/3
  Demux3/3 -> " denormalizing reference4"/3(soot_norm)
  In4/1 -> Demux3/1
  " denormalizing reference4"/2(NOX) -> Mux3/2
  " denormalizing reference4"/1(IMEP) -> Mux3/1
  Demux3/1 -> " denormalizing reference4"/1(IMEP_norm)
  Demux3/4 -> " denormalizing reference4"/4(MPRR_norm)
  Demux3/2 -> " denormalizing reference4"/2(NOX_norm)
  " denormalizing reference4"/4(MPRR) -> Mux3/4
  Mux/1 -> Node_0/1
  Mux1/1 -> Node_1/1
  Mux2/1 -> Node_2/1
  Mux3/1 -> Node_3/1

== system pi_OfflineRL_H2DF_2023a/main_C2C_RL/RL_Controller/RL_Controller_ifAction/RL_Controller_PPO1/Subsystem ==
  note: 1:TD3
      | 2:PPO
  Refernce : Inport
  Outputs : Inport  Port=2
  LSTM States : Inport  Port=3
  Enable : Inport  Port=4
  If : If
  If Action Subsystem : Subsystem  TreatAsAtomicUnit=on
  If Action Subsystem1 : Subsystem  TreatAsAtomicUnit=on
  Merge : Merge
  Selector3 : Selector  IndexOptions=Index vector (dialog)  Indices=[5:8]  OutputSizes=1
  Observation : Outport
  wires:
  Selector3/1 -> If Action Subsystem/1(Reference)
  Refernce/1 -> Selector3/1
  Outputs/1 -> If Action Subsystem/2(Outputs)
  Enable/1 -> If Action Subsystem/4(Enable), If/1
  If/1 -> If Action Subsystem/Action
  If/2 -> If Action Subsystem1/Action
  If Action Subsystem/1(observations) -> Merge/1
  If Action Subsystem1/1(observations) -> Merge/2
  Merge/1 -> Observation/1
  LSTM States/1 -> If Action Subsystem/3(LSTM States)

== system pi_OfflineRL_H2DF_2023a/main_C2C_RL/RL_Controller/RL_Controller_ifAction/RL_Controller_PPO2/Subsystem ==
  note: 1:TD3
      | 2:PPO
  Refernce : Inport
  Outputs : Inport  Port=2
  LSTM States : Inport  Port=3
  Enable : Inport  Port=4
  If : If
  If Action Subsystem : Subsystem  TreatAsAtomicUnit=on
  If Action Subsystem1 : Subsystem  TreatAsAtomicUnit=on
  Merge : Merge
  Selector3 : Selector  IndexOptions=Index vector (dialog)  Indices=[5:8]  OutputSizes=1
  Observation : Outport
  wires:
  Selector3/1 -> If Action Subsystem/1(Reference)
  Refernce/1 -> Selector3/1
  Outputs/1 -> If Action Subsystem/2(Outputs)
  Enable/1 -> If Action Subsystem/4(Enable), If/1
  If/1 -> If Action Subsystem/Action
  If/2 -> If Action Subsystem1/Action
  If Action Subsystem/1(observations) -> Merge/1
  If Action Subsystem1/1(observations) -> Merge/2
  Merge/1 -> Observation/1
  LSTM States/1 -> If Action Subsystem/3(LSTM States)

== system pi_OfflineRL_H2DF_2023a/main_C2C_RL/RL_Controller/RL_Controller_ifAction/RL_Controller_PPO3/Subsystem ==
  note: 1:TD3
      | 2:PPO
  Refernce : Inport
  Outputs : Inport  Port=2
  LSTM States : Inport  Port=3
  Enable : Inport  Port=4
  If : If
  If Action Subsystem : Subsystem  TreatAsAtomicUnit=on
  If Action Subsystem1 : Subsystem  TreatAsAtomicUnit=on
  Merge : Merge
  Selector3 : Selector  IndexOptions=Index vector (dialog)  Indices=[5:8]  OutputSizes=1
  Observation : Outport
  wires:
  Selector3/1 -> If Action Subsystem/1(Reference)
  Refernce/1 -> Selector3/1
  Outputs/1 -> If Action Subsystem/2(Outputs)
  Enable/1 -> If Action Subsystem/4(Enable), If/1
  If/1 -> If Action Subsystem/Action
  If/2 -> If Action Subsystem1/Action
  If Action Subsystem/1(observations) -> Merge/1
  If Action Subsystem1/1(observations) -> Merge/2
  Merge/1 -> Observation/1
  LSTM States/1 -> If Action Subsystem/3(LSTM States)

== system pi_OfflineRL_H2DF_2023a/main_C2C_RL/RL_Controller/RL_Controller_ifAction/RL_Controller_PPO4/Subsystem ==
  note: 1:TD3
      | 2:PPO
  Refernce : Inport
  Outputs : Inport  Port=2
  LSTM States : Inport  Port=3
  Enable : Inport  Port=4
  If : If
  If Action Subsystem : Subsystem  TreatAsAtomicUnit=on
  If Action Subsystem1 : Subsystem  TreatAsAtomicUnit=on
  Merge : Merge
  Selector3 : Selector  IndexOptions=Index vector (dialog)  Indices=[5:8]  OutputSizes=1
  Observation : Outport
  wires:
  Selector3/1 -> If Action Subsystem/1(Reference)
  Refernce/1 -> Selector3/1
  Outputs/1 -> If Action Subsystem/2(Outputs)
  Enable/1 -> If Action Subsystem/4(Enable), If/1
  If/1 -> If Action Subsystem/Action
  If/2 -> If Action Subsystem1/Action
  If Action Subsystem/1(observations) -> Merge/1
  If Action Subsystem1/1(observations) -> Merge/2
  Merge/1 -> Observation/1
  LSTM States/1 -> If Action Subsystem/3(LSTM States)

== system pi_OfflineRL_H2DF_2023a/main_C2C_RL/RL_Controller/RL_Controller_ifAction/RL_Controller_PPO5/Subsystem ==
  note: 1:TD3
      | 2:PPO
  Refernce : Inport
  Outputs : Inport  Port=2
  LSTM States : Inport  Port=3
  Enable : Inport  Port=4
  If : If
  If Action Subsystem : Subsystem  TreatAsAtomicUnit=on
  If Action Subsystem1 : Subsystem  TreatAsAtomicUnit=on
  Merge : Merge
  Selector3 : Selector  IndexOptions=Index vector (dialog)  Indices=[5:8]  OutputSizes=1
  Observation : Outport
  wires:
  Selector3/1 -> If Action Subsystem/1(Reference)
  Refernce/1 -> Selector3/1
  Outputs/1 -> If Action Subsystem/2(Outputs)
  Enable/1 -> If Action Subsystem/4(Enable), If/1
  If/1 -> If Action Subsystem/Action
  If/2 -> If Action Subsystem1/Action
  If Action Subsystem/1(observations) -> Merge/1
  If Action Subsystem1/1(observations) -> Merge/2
  Merge/1 -> Observation/1
  LSTM States/1 -> If Action Subsystem/3(LSTM States)

== system pi_OfflineRL_H2DF_2023a/main_C2C_RL/RL_Controller/RL_Controller_ifAction/RL_Controller_PPO6/Subsystem ==
  note: 1:TD3
      | 2:PPO
  Refernce : Inport
  Outputs : Inport  Port=2
  LSTM States : Inport  Port=3
  Enable : Inport  Port=4
  If : If
  If Action Subsystem : Subsystem  TreatAsAtomicUnit=on
  If Action Subsystem1 : Subsystem  TreatAsAtomicUnit=on
  Merge : Merge
  Selector3 : Selector  IndexOptions=Index vector (dialog)  Indices=[5:8]  OutputSizes=1
  Observation : Outport
  wires:
  Selector3/1 -> If Action Subsystem/1(Reference)
  Refernce/1 -> Selector3/1
  Outputs/1 -> If Action Subsystem/2(Outputs)
  Enable/1 -> If Action Subsystem/4(Enable), If/1
  If/1 -> If Action Subsystem/Action
  If/2 -> If Action Subsystem1/Action
  If Action Subsystem/1(observations) -> Merge/1
  If Action Subsystem1/1(observations) -> Merge/2
  Merge/1 -> Observation/1
  LSTM States/1 -> If Action Subsystem/3(LSTM States)

== system pi_OfflineRL_H2DF_2023a/main_C2C_RL/RL_Controller/RL_Controller_ifAction/RL_Controller_PPO7/Subsystem ==
  note: 1:TD3
      | 2:PPO
  Refernce : Inport
  Outputs : Inport  Port=2
  LSTM States : Inport  Port=3
  Enable : Inport  Port=4
  If : If
  If Action Subsystem : Subsystem  TreatAsAtomicUnit=on
  If Action Subsystem1 : Subsystem  TreatAsAtomicUnit=on
  Merge : Merge
  Selector3 : Selector  IndexOptions=Index vector (dialog)  Indices=[5:8]  OutputSizes=1
  Observation : Outport
  wires:
  Selector3/1 -> If Action Subsystem/1(Reference)
  Refernce/1 -> Selector3/1
  Outputs/1 -> If Action Subsystem/2(Outputs)
  Enable/1 -> If Action Subsystem/4(Enable), If/1
  If/1 -> If Action Subsystem/Action
  If/2 -> If Action Subsystem1/Action
  If Action Subsystem/1(observations) -> Merge/1
  If Action Subsystem1/1(observations) -> Merge/2
  Merge/1 -> Observation/1
  LSTM States/1 -> If Action Subsystem/3(LSTM States)

== system pi_OfflineRL_H2DF_2023a/main_C2C_RL/RL_Controller/RL_Controller_ifAction/RL_Controller_PPO8/Subsystem ==
  note: 1:TD3
      | 2:PPO
  Refernce : Inport
  Outputs : Inport  Port=2
  LSTM States : Inport  Port=3
  Enable : Inport  Port=4
  If : If
  If Action Subsystem : Subsystem  TreatAsAtomicUnit=on
  If Action Subsystem1 : Subsystem  TreatAsAtomicUnit=on
  Merge : Merge
  Selector3 : Selector  IndexOptions=Index vector (dialog)  Indices=[5:8]  OutputSizes=1
  Observation : Outport
  wires:
  Selector3/1 -> If Action Subsystem/1(Reference)
  Refernce/1 -> Selector3/1
  Outputs/1 -> If Action Subsystem/2(Outputs)
  Enable/1 -> If Action Subsystem/4(Enable), If/1
  If/1 -> If Action Subsystem/Action
  If/2 -> If Action Subsystem1/Action
  If Action Subsystem/1(observations) -> Merge/1
  If Action Subsystem1/1(observations) -> Merge/2
  Merge/1 -> Observation/1
  LSTM States/1 -> If Action Subsystem/3(LSTM States)

== system pi_OfflineRL_H2DF_2023a/main_C2C_RL/post_processing/Subsystem1/Subsystem/ denormalizing reference1 ==
  IMEP_norm : Inport
  NOX_norm : Inport  Port=2
  soot_norm : Inport  Port=3
  MPRR_norm : Inport  Port=4
  Constant : Constant  Value=C2C_NMPC.Normalization.outputs.mean(1)
  Constant1 : Constant  Value=C2C_NMPC.Normalization.outputs.mean(2)
  Constant2 : Constant  Value=C2C_NMPC.Normalization.outputs.mean(3)
  Constant3 : Constant  Value=C2C_NMPC.Normalization.outputs.mean(4)
  Gain : Gain  Gain=C2C_NMPC.Normalization.outputs.std(1)
  Gain1 : Gain  Gain=C2C_NMPC.Normalization.outputs.std(2)
  Gain2 : Gain  Gain=C2C_NMPC.Normalization.outputs.std(3)
  Gain3 : Gain  Gain=C2C_NMPC.Normalization.outputs.std(4)
  Sum{1..3,5} (4 alike) : Sum  Inputs=|++
  IMEP : Outport
  NOX : Outport  Port=2
  soot : Outport  Port=3
  MPRR : Outport  Port=4
  wires:
  Gain/1 -> Sum5/1
  IMEP_norm/1 -> Gain/1
  Constant/1 -> Sum5/2
  Sum5/1 -> IMEP/1
  Gain1/1 -> Sum1/1
  Constant1/1 -> Sum1/2
  NOX_norm/1 -> Gain1/1
  Sum1/1 -> NOX/1
  Gain2/1 -> Sum2/1
  Constant2/1 -> Sum2/2
  soot_norm/1 -> Gain2/1
  Sum2/1 -> soot/1
  Gain3/1 -> Sum3/1
  Constant3/1 -> Sum3/2
  MPRR_norm/1 -> Gain3/1
  Sum3/1 -> MPRR/1

== system pi_OfflineRL_H2DF_2023a/main_C2C_RL/post_processing/Subsystem1/Subsystem/ denormalizing reference2 ==
  IMEP_norm : Inport
  NOX_norm : Inport  Port=2
  soot_norm : Inport  Port=3
  MPRR_norm : Inport  Port=4
  Constant : Constant  Value=C2C_NMPC.Normalization.outputs.mean(1)
  Constant1 : Constant  Value=C2C_NMPC.Normalization.outputs.mean(2)
  Constant2 : Constant  Value=C2C_NMPC.Normalization.outputs.mean(3)
  Constant3 : Constant  Value=C2C_NMPC.Normalization.outputs.mean(4)
  Gain : Gain  Gain=C2C_NMPC.Normalization.outputs.std(1)
  Gain1 : Gain  Gain=C2C_NMPC.Normalization.outputs.std(2)
  Gain2 : Gain  Gain=C2C_NMPC.Normalization.outputs.std(3)
  Gain3 : Gain  Gain=C2C_NMPC.Normalization.outputs.std(4)
  Sum{1..3,5} (4 alike) : Sum  Inputs=|++
  IMEP : Outport
  NOX : Outport  Port=2
  soot : Outport  Port=3
  MPRR : Outport  Port=4
  wires:
  Gain/1 -> Sum5/1
  IMEP_norm/1 -> Gain/1
  Constant/1 -> Sum5/2
  Sum5/1 -> IMEP/1
  Gain1/1 -> Sum1/1
  Constant1/1 -> Sum1/2
  NOX_norm/1 -> Gain1/1
  Sum1/1 -> NOX/1
  Gain2/1 -> Sum2/1
  Constant2/1 -> Sum2/2
  soot_norm/1 -> Gain2/1
  Sum2/1 -> soot/1
  Gain3/1 -> Sum3/1
  Constant3/1 -> Sum3/2
  MPRR_norm/1 -> Gain3/1
  Sum3/1 -> MPRR/1

== system pi_OfflineRL_H2DF_2023a/main_C2C_RL/post_processing/Subsystem1/Subsystem/ denormalizing reference3 ==
  IMEP_norm : Inport
  NOX_norm : Inport  Port=2
  soot_norm : Inport  Port=3
  MPRR_norm : Inport  Port=4
  Constant : Constant  Value=C2C_NMPC.Normalization.outputs.mean(1)
  Constant1 : Constant  Value=C2C_NMPC.Normalization.outputs.mean(2)
  Constant2 : Constant  Value=C2C_NMPC.Normalization.outputs.mean(3)
  Constant3 : Constant  Value=C2C_NMPC.Normalization.outputs.mean(4)
  Gain : Gain  Gain=C2C_NMPC.Normalization.outputs.std(1)
  Gain1 : Gain  Gain=C2C_NMPC.Normalization.outputs.std(2)
  Gain2 : Gain  Gain=C2C_NMPC.Normalization.outputs.std(3)
  Gain3 : Gain  Gain=C2C_NMPC.Normalization.outputs.std(4)
  Sum{1..3,5} (4 alike) : Sum  Inputs=|++
  IMEP : Outport
  NOX : Outport  Port=2
  soot : Outport  Port=3
  MPRR : Outport  Port=4
  wires:
  Gain/1 -> Sum5/1
  IMEP_norm/1 -> Gain/1
  Constant/1 -> Sum5/2
  Sum5/1 -> IMEP/1
  Gain1/1 -> Sum1/1
  Constant1/1 -> Sum1/2
  NOX_norm/1 -> Gain1/1
  Sum1/1 -> NOX/1
  Gain2/1 -> Sum2/1
  Constant2/1 -> Sum2/2
  soot_norm/1 -> Gain2/1
  Sum2/1 -> soot/1
  Gain3/1 -> Sum3/1
  Constant3/1 -> Sum3/2
  MPRR_norm/1 -> Gain3/1
  Sum3/1 -> MPRR/1

== system pi_OfflineRL_H2DF_2023a/main_C2C_RL/post_processing/Subsystem1/Subsystem/ denormalizing reference4 ==
  IMEP_norm : Inport
  NOX_norm : Inport  Port=2
  soot_norm : Inport  Port=3
  MPRR_norm : Inport  Port=4
  Constant : Constant  Value=C2C_NMPC.Normalization.outputs.mean(1)
  Constant1 : Constant  Value=C2C_NMPC.Normalization.outputs.mean(2)
  Constant2 : Constant  Value=C2C_NMPC.Normalization.outputs.mean(3)
  Constant3 : Constant  Value=C2C_NMPC.Normalization.outputs.mean(4)
  Gain : Gain  Gain=C2C_NMPC.Normalization.outputs.std(1)
  Gain1 : Gain  Gain=C2C_NMPC.Normalization.outputs.std(2)
  Gain2 : Gain  Gain=C2C_NMPC.Normalization.outputs.std(3)
  Gain3 : Gain  Gain=C2C_NMPC.Normalization.outputs.std(4)
  Sum{1..3,5} (4 alike) : Sum  Inputs=|++
  IMEP : Outport
  NOX : Outport  Port=2
  soot : Outport  Port=3
  MPRR : Outport  Port=4
  wires:
  Gain/1 -> Sum5/1
  IMEP_norm/1 -> Gain/1
  Constant/1 -> Sum5/2
  Sum5/1 -> IMEP/1
  Gain1/1 -> Sum1/1
  Constant1/1 -> Sum1/2
  NOX_norm/1 -> Gain1/1
  Sum1/1 -> NOX/1
  Gain2/1 -> Sum2/1
  Constant2/1 -> Sum2/2
  soot_norm/1 -> Gain2/1
  Sum2/1 -> soot/1
  Gain3/1 -> Sum3/1
  Constant3/1 -> Sum3/2
  MPRR_norm/1 -> Gain3/1
  Sum3/1 -> MPRR/1
